simulink model "positioncontrol"  (R2019a)
settings: Solver=ode3  StartTime=0.0  StopTime=100.0  RelTol=1e-3
values from neighbouring files (symbols this model uses):
  th_0 = (3*pi)/180    (= 0.0523598775598)    [ejercicio2.m]
undefined symbols (not defined in the file or in its folder): DiscIntNeverNeededParam, refx, refy
libraries: fuzblock x1, simulink x1
settings Model: Creator=pizarro  LastModifiedBy=tromp
settings DataIOCC: ReturnWorkspaceOutputs=off

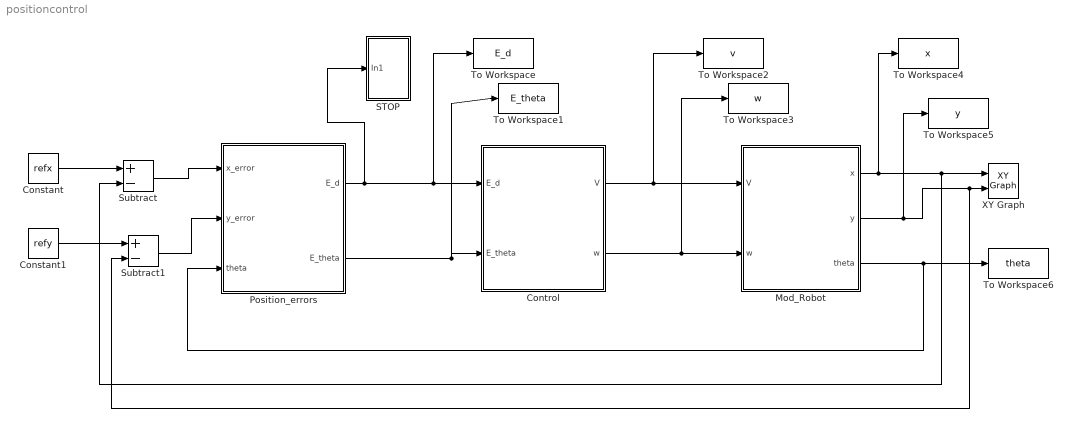
== system positioncontrol ==
  Constant : Constant  Value=refx
  Constant1 : Constant  Value=refy
  Control : Subsystem
  Mod_Robot : Subsystem
  Position_errors : Subsystem
  STOP : Subsystem
  Subtract : Sum  Inputs=+-
  Subtract1 : Sum  Inputs=+-
  To Workspace : ToWorkspace  VariableName=E_d  SaveFormat=Structure With Time  SampleTime=-1
  To Workspace1 : ToWorkspace  VariableName=E_theta  SaveFormat=Structure With Time  SampleTime=-1
  To Workspace2 : ToWorkspace  VariableName=v  SaveFormat=Structure With Time  SampleTime=-1
  To Workspace3 : ToWorkspace  VariableName=w  SaveFormat=Structure With Time  SampleTime=-1
  To Workspace4 : ToWorkspace  VariableName=x  SaveFormat=Structure With Time  SampleTime=-1
  To Workspace5 : ToWorkspace  VariableName=y  SaveFormat=Structure With Time  SampleTime=-1
  To Workspace6 : ToWorkspace  VariableName=theta  SaveFormat=Structure With Time  SampleTime=-1
  XY Graph : simulink/Sinks/XY Graph  xmin=-10  xmax=10  ymin=-10  ymax=10  st=-1
  wires:
  Position_errors/2(E_theta) -> To Workspace1/1, Control/2(E_theta)
  Position_errors/1(E_d) -> STOP/1(In1), To Workspace/1, Control/1(E_d)
  Control/1(V) -> To Workspace2/1, Mod_Robot/1(V)
  Control/2(w) -> To Workspace3/1, Mod_Robot/2(w)
  Mod_Robot/1(x) -> To Workspace4/1, Subtract/2, XY Graph/1
  Mod_Robot/2(y) -> To Workspace5/1, Subtract1/2, XY Graph/2
  Mod_Robot/3("theta ") -> Position_errors/3(theta), To Workspace6/1
  Constant/1 -> Subtract/1
  Constant1/1 -> Subtract1/1
  Subtract/1 -> Position_errors/1(x_error)
  Subtract1/1 -> Position_errors/2(y_error)

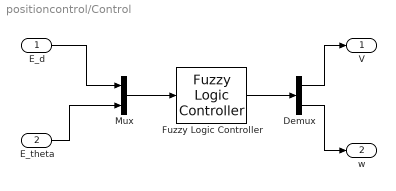
== system positioncontrol/Control ==
  E_d : Inport
  E_theta : Inport  Port=2
  Demux : Demux  Outputs=2
  Fuzzy Logic Controller : fuzblock/Fuzzy Logic  Controller  FIS='controladorBorrosoSimple.fis'  OutputSampleNumber=101  DataType=double  FuzzifiedInputs=off  RuleFiringStrengths=off  RuleOutputs=off  AggregatedOutputs=off  SimulateUsing=Interpreted execution  OutOfRangeInputValueMessage=warning  NoRuleFiredMessage=warning  EmptyOutputFuzzySetMessage=warning
  Mux : Mux  Inputs=2
  V : Outport
  w : Outport  Port=2
  wires:
  E_d/1 -> Mux/1
  E_theta/1 -> Mux/2
  Mux/1 -> Fuzzy Logic Controller/1
  Fuzzy Logic Controller/1 -> Demux/1
  Demux/1 -> V/1
  Demux/2 -> w/1

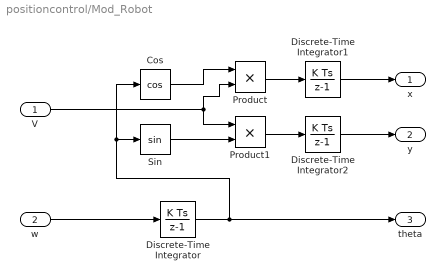
== system positioncontrol/Mod_Robot ==
  V : Inport
  w : Inport  Port=2
  Cos : Trigonometry  Operator=cos
  Discrete-Time Integrator : DiscreteIntegrator  InitialCondition=th_0  SampleTime=0.01  ICPrevOutput=DiscIntNeverNeededParam  ICPrevScaledInput=DiscIntNeverNeededParam
  Discrete-Time Integrator1 : DiscreteIntegrator  SampleTime=0.01  ICPrevOutput=DiscIntNeverNeededParam  ICPrevScaledInput=DiscIntNeverNeededParam
  Discrete-Time Integrator2 : DiscreteIntegrator  SampleTime=0.01  ICPrevOutput=DiscIntNeverNeededParam  ICPrevScaledInput=DiscIntNeverNeededParam
  Product : Product
  Product1 : Product
  Sin : Trigonometry
  x : Outport
  y : Outport  Port=2
  "theta " : Outport  Port=3
  wires:
  Discrete-Time Integrator/1 -> "theta "/1, Cos/1, Sin/1
  Cos/1 -> Product/1
  Product1/1 -> Discrete-Time Integrator2/1
  Product/1 -> Discrete-Time Integrator1/1
  Discrete-Time Integrator1/1 -> x/1
  V/1 -> Product/2, Product1/1
  Discrete-Time Integrator2/1 -> y/1
  Sin/1 -> Product1/2
  w/1 -> Discrete-Time Integrator/1

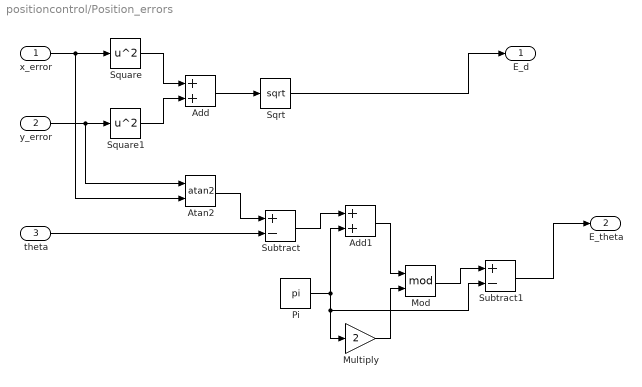
== system positioncontrol/Position_errors ==
  x_error : Inport
  y_error : Inport  Port=2
  theta : Inport  Port=3
  Add : Sum
  Add1 : Sum
  Atan2 : Trigonometry  Operator=atan2
  Mod : Math  Operator=mod  SaturateOnIntegerOverflow=on
  Multiply : Gain  Gain=2
  Pi : Constant  Value=pi  OutDataTypeStr=Inherit: Inherit via back propagation
  Sqrt : Sqrt  SaturateOnIntegerOverflow=on
  Square : Math  Operator=square  SaturateOnIntegerOverflow=on
  Square1 : Math  Operator=square  SaturateOnIntegerOverflow=on
  Subtract : Sum  Inputs=+-
  Subtract1 : Sum  Inputs=+-
  E_d : Outport
  E_theta : Outport  Port=2
  wires:
  Sqrt/1 -> E_d/1
  y_error/1 -> Atan2/1, Square1/1
  x_error/1 -> Atan2/2, Square/1
  Square1/1 -> Add/2
  Add/1 -> Sqrt/1
  Square/1 -> Add/1
  Atan2/1 -> Subtract/1
  theta/1 -> Subtract/2
  Subtract/1 -> Add1/1
  Pi/1 -> Subtract1/2, Multiply/1, Add1/2
  Multiply/1 -> Mod/2
  Add1/1 -> Mod/1
  Mod/1 -> Subtract1/1
  Subtract1/1 -> E_theta/1

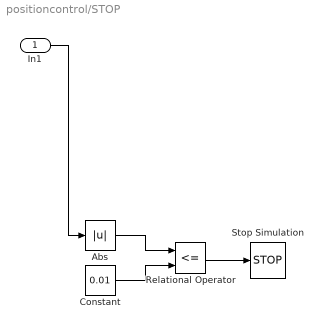
== system positioncontrol/STOP ==
  In1 : Inport
  Abs : Abs
  Constant : Constant  Value=0.01
  Relational Operator : RelationalOperator  Operator=<=  OutDataTypeStr=boolean  RndMeth=Simplest
  Stop Simulation : Stop
  wires:
  Abs/1 -> Relational Operator/1
  Constant/1 -> Relational Operator/2
  Relational Operator/1 -> Stop Simulation/1
  In1/1 -> Abs/1
